simulink model "MTDC_MODEL"  (R2021a)
settings: Solver=ode1  StartTime=0.0  StopTime=3  FixedStep=2e-5  MaxStep=1e-5  RelTol=1e-5  EnableMultiTasking=on
InitFcn:
  | tau_iac=ts_G_iac/4;                                         %Current loop speed
  | wAC=1/tau_iac;                                              %Frequency
  | L1AC=wAC/s;                                                 %Open loop IMC (L) transfer function to obtain a first order after closing the loop
  | Kp_AC=wAC*(Lg_1+La_1/2);                                    %Proportional constant of the controller
  | Ki_AC=wAC*(Rg_1+Ra_1/2);                                    %Integral constant of the controller
  | C_IMC_AC=(Kp_AC*s+Ki_AC)/s;                                 %IMC designed PI controller transfer function
  | TAC=minreal((C_IMC_AC)*G_iac/(1+(C_IMC_AC)*G_iac));         %Closed loop transfer function
  | 
  | tau_Pac=ts_G_P/4;
  | D = TAC*U_ll1;
  | [C_pi,info] = pidtune(D,'PI',1/tau_Pac);
  | Ki_P = C_pi.Ki;
  | 
  | tau_Qac=ts_G_Q/4;
  | [C_piq,info] = pidtune(D,'PI',1/tau_Qac);
  | Ki_Q = C_piq.Ki;
  | 
  | 
  | tau_isum=ts_G_isum/4;                                        %Current loop speed
  | wsum=1/tau_isum;                                             %Frequency
  | L1AC=wsum/s;                                                 %Open loop IMC (L) transfer function to obtain a first order after closing the loop
  | Kp_sum=wsum*(2*La_1);                                        %Proportional constant of the controller
  | Ki_sum=wsum*(2*Ra_1);                                        %Integral constant of the controller
  | C_IMC_sum=(Kp_sum*s+Ki_sum)/s;                               %IMC designed PI controller transfer function
  | 
  | Kp_sum_PR = wc*(2*La_1);
  | Ki_sum_PR = wc*(2*Ra_1);
  | PR = (Kp_sum_PR*s^2 + 2*wc*(Kp_sum_PR+Ki_sum_PR)*s +Kp_sum_PR*w0^2)/(s^2+2*wc*s+w0^2);
  | 
  | 
  | %Energy reference for a converter arm (sum of all the submodule energies)
  | ArmEnergyRef=1/2*Carm*ArmVoltageRef^2;                      %Energy reference for a converter leg
  | LegEnergy=ArmEnergyRef*2;                                   %References for the controllers (DC side)
  | TotalEnergyRef=ArmEnergyRef*6;                              %Reference of the total energy of the converter
  | EnergyDiffabRef=0;                                          %Reference for the energy difference between legs a and b
  | EnergyDiffacRef=0;                                          %Reference for the energy difference between legs b and c
  | 
  | %References for the controllers (AC side)
  | EnergyDiffUpLowRefa=0;                                      %Reference for the energy difference upper and lower arms of phase a
  | EnergyDiffUpLowRefb=0;                                      %Reference for the energy difference upper and lower arms of phase b
  | EnergyDiffUpLowRefc=0;                                      %Reference for the energy difference upper and lower arms of phase c
  |                                                             %Controller design
  | Kpenergy=50;                                                %Proportional gain
  | Kienergy=20;                                                %Integral gain
  | 
  | Kpenergyt=50;                                               %Proportional gain
  | Kienergyt=20;                                               %Integral gain
  | 
  | Q=3;
  | wn=50*2*pi;                                                 %Frequency to eliminate 50 Hz
  | N_50 = tf([1 0 wn^2],[1 2*wn/Q wn^2]);                       %Notch filter 1 design
  | wn=100*2*pi;                                                %Frequency to eliminate 100 Hz
  | N_100 = tf([1 0 wn^2],[1 2*wn/Q wn^2]);                      %Notch filter 2 design
  | Notch=N_50*N_100;                                            %Combination of both notch filters
  | 
  | Ibasedc1= 1000e6/640e3;                 %Nominal current peak DC
  | IsaturationinnerDC1=1.1*Ibasedc1/3;  %Saturation of the DC inner current
  | IsaturationinnerAC1=0.45*Ibasedc1/3; %0.45  %Saturation of the inner current (why edu used 10% - FYI I changed it to 45%)
  | 
  | 
  | ... (+30 lines)
values from neighbouring files (symbols this model uses):
  ArmVoltageRef = 640e3    (= 640000)    [MMC_PARAMETERS.m]
  Cap = 9.5e-3    (= 0.0095)    [MMC_PARAMETERS.m]
  Carm = Cap/N    (= 2.375e-05)    [MMC_PARAMETERS.m]
  f_grid = 50    [MMC_PARAMETERS.m]
  La_1 = 0.15*Zbase_1/2/pi/50    (= 0.0488923985178)    [MMC_PARAMETERS.m]
  Lg_1 = 0.18*Zbase_1/2/pi/50    (= 0.0586708782214)    [MMC_PARAMETERS.m]
  N = 400    [MMC_PARAMETERS.m]
  Ra_1 = 0.01*Zbase_1    (= 1.024)    [MMC_PARAMETERS.m]
  Rg_1 = 0.005*Zbase_1    (= 0.512)    [MMC_PARAMETERS.m]
  S_1 = 1000e6    (= 1000000000)    [MMC_PARAMETERS.m]
  U_ll1 = 320e3    (= 320000)    [MMC_PARAMETERS.m]
  Vdc = 640e3    (= 640000)    [MMC_PARAMETERS.m]
  Vpeak_d1 = U_pnpeak1    [MMC_PARAMETERS.m]
  w0 = 2*pi*50    (= 314.159265359)    [MMC_PARAMETERS.m]
undefined symbols (not defined in the file or in its folder): Kp_Pac, lenght
libraries: spsSeriesRLCBranchLib x80, spsCurrentMeasurementLib x64, spsControlledVoltageSourceLib x36, pid_lib x32, spsVoltageMeasurementLib x32, spsControlledCurrentSourceLib x24, spsParallelRLCBranchLib x20, spsGroundLib x10, powerlib_extras x4, spsDCVoltageSourceLib x4, spspowerguiLib x1
(part 4 of 9)

== system MTDC_MODEL/GRID1+MMC1/Equivalent arm upper-b ==
  note: Power_ub
  vub : Inport
  Controlled Current Source : spsControlledCurrentSourceLib/Controlled Current Source  Initialize=on  Source_Type=AC  Amplitude=0  Phase=0  Frequency=0  Measurements=None
  Controlled Voltage Source7 : spsControlledVoltageSourceLib/Controlled Voltage Source  Initialize=on  Source_Type=AC  Amplitude=Vdc/2  Phase=0  Frequency=0  Measurements=None
  Current Measurement4 : spsCurrentMeasurementLib/Current Measurement  PhasorSimulation=off  OutputType=Complex  PSBequivalent=0
  Divide1 : Product  Inputs=**
  Divide2 : Product  Inputs=*/
  Filtered Upper arm A instananeous power1 : Scope
  Gain : Gain  Gain=1e6
  Series RLC Branch2 : spsSeriesRLCBranchLib/Series RLC Branch  LConnTagsString=__new0  RConnTagsString=__new0  BranchType=C  Resistance=Ra_1  Inductance=La_1  SetiL0=on  InitialCurrent=0  Capacitance=Cap/N  Setx0=on  InitialVoltage=640e3  Measurements=None
  Transfer Fcn : TransferFcn  Denominator=[1 1]
  Upper arm A instananeous power : Scope
  Voltage Measurement : spsVoltageMeasurementLib/Voltage Measurement  PhasorSimulation=off  OutputType=Complex  PSBequivalent=0
  Conn1 : PMIOPort  Side=Right
  Conn2 : PMIOPort  Port=2  Side=Left
  v_sum_ub : Outport
  wires:
  vub/1 -> Divide1/1, Controlled Voltage Source7/1  "vub"
  Voltage Measurement/1 -> v_sum_ub/1, Divide2/2
  Divide2/1 -> Controlled Current Source/1
  Divide1/1 -> Upper arm A instananeous power/1, Transfer Fcn/1, Divide2/1
  Current Measurement4/1 -> Divide1/2  "iub"
  Transfer Fcn/1 -> Gain/1
  Gain/1 -> Filtered Upper arm A instananeous power1/1
  connections:
  Controlled Voltage Source7/RConn1 -- Conn1/RConn1
  Voltage Measurement/LConn1 -- Series RLC Branch2/LConn1 -- Controlled Current Source/RConn1
  Controlled Current Source/LConn1 -- Series RLC Branch2/RConn1 -- Voltage Measurement/LConn2
  Current Measurement4/LConn1 -- Controlled Voltage Source7/LConn1
  Conn2/RConn1 -- Current Measurement4/RConn1

== system MTDC_MODEL/GRID1+MMC1/Equivalent arm upper-c ==
  note: Power_uc
  vuc : Inport
  Controlled Current Source : spsControlledCurrentSourceLib/Controlled Current Source  Initialize=on  Source_Type=AC  Amplitude=0  Phase=0  Frequency=0  Measurements=None
  Controlled Voltage Source7 : spsControlledVoltageSourceLib/Controlled Voltage Source  Initialize=on  Source_Type=AC  Amplitude=Vdc/2  Phase=0  Frequency=0  Measurements=None
  Current Measurement4 : spsCurrentMeasurementLib/Current Measurement  PhasorSimulation=off  OutputType=Complex  PSBequivalent=0
  Divide1 : Product  Inputs=**
  Divide2 : Product  Inputs=*/
  Filtered Upper arm A instananeous power1 : Scope
  Gain : Gain  Gain=1e6
  Series RLC Branch2 : spsSeriesRLCBranchLib/Series RLC Branch  LConnTagsString=__new0  RConnTagsString=__new0  BranchType=C  Resistance=Ra_1  Inductance=La_1  SetiL0=on  InitialCurrent=0  Capacitance=Cap/N  Setx0=on  InitialVoltage=640e3  Measurements=None
  Transfer Fcn : TransferFcn  Denominator=[1 1]
  Upper arm A instananeous power : Scope
  Voltage Measurement : spsVoltageMeasurementLib/Voltage Measurement  PhasorSimulation=off  OutputType=Complex  PSBequivalent=0
  Conn1 : PMIOPort  Side=Right
  Conn2 : PMIOPort  Port=2  Side=Left
  v_sum_uc : Outport
  wires:
  vuc/1 -> Divide1/1, Controlled Voltage Source7/1  "vuc"
  Voltage Measurement/1 -> v_sum_uc/1, Divide2/2
  Divide2/1 -> Controlled Current Source/1
  Divide1/1 -> Upper arm A instananeous power/1, Transfer Fcn/1, Divide2/1
  Current Measurement4/1 -> Divide1/2  "iuc"
  Transfer Fcn/1 -> Gain/1
  Gain/1 -> Filtered Upper arm A instananeous power1/1
  connections:
  Controlled Voltage Source7/RConn1 -- Conn1/RConn1
  Voltage Measurement/LConn1 -- Series RLC Branch2/LConn1 -- Controlled Current Source/RConn1
  Controlled Current Source/LConn1 -- Series RLC Branch2/RConn1 -- Voltage Measurement/LConn2
  Current Measurement4/LConn1 -- Controlled Voltage Source7/LConn1
  Conn2/RConn1 -- Current Measurement4/RConn1

== system MTDC_MODEL/GRID1+MMC1/Feedforward calculation ==
  vzabc : Inport
  isabc : Inport  Port=2
  Demux1 : Demux  Outputs=3
  First order filter1 : Subsystem
  Mux2 : Mux  Inputs=2
  PI10 : TransferFcn  Numerator=[Notch.num{1}]  Denominator=[Notch.den{1}]
  PI9 : TransferFcn  Numerator=[Notch.num{1}]  Denominator=[Notch.den{1}]
  Product5 : Product
  Scope3 : Scope
  Sum15 : Sum  Inputs=|+-
  Sum39 : Sum  Inputs=|+-
  Sum5 : Sum  Inputs=+++
  Pt : Outport  VectorParamsAs1DForOutWhenUnconnected=off
  Pab : Outport  Port=2  VectorParamsAs1DForOutWhenUnconnected=off
  Pac : Outport  Port=3  VectorParamsAs1DForOutWhenUnconnected=off
  wires:
  Demux1/3 -> Sum39/2, Sum5/3
  Demux1/2 -> Sum15/2, Sum5/2
  Demux1/1 -> Sum15/1, Sum39/1, Sum5/1
  vzabc/1 -> Product5/1
  Sum15/1 -> Pab/1, PI9/1  "Pa-Pb"
  Sum39/1 -> Pac/1, PI10/1  "Pb-Pc"
  Product5/1 -> First order filter1/1(In1)
  First order filter1/1(Out1) -> Demux1/1
  isabc/1 -> Product5/2
  Sum5/1 -> Pt/1
  Mux2/1 -> Scope3/1
  PI9/1 -> Mux2/1
  PI10/1 -> Mux2/2

== system MTDC_MODEL/GRID1+MMC1/Grid3 ==
  Constant : Constant
  Constant1 : Constant  Value=f_grid
  Constant{2,5..7,20} (5 alike) : Constant  Value=0
  Constant21 : Constant  Value=-2*pi/3
  Constant22 : Constant  Value=2*pi/3
  Constant8 : Constant  Value=2*pi/3
  Constant9 : Constant  Value=-2*pi/3
  Gain1 : Gain  Gain=2*pi
  Gain{2..3,6,8} (4 alike) : Gain  Gain=Vpeak_d1
  Gain4 : Gain  Gain=0
  Gain5 : Gain  Gain=0
  Gain7 : Gain  Gain=0
  Integrator{1..3,8..10} (6 alike) : Integrator
  Sum{1..12} (12 alike) : Sum  Inputs=|++
  Trigonometric Function{1..3,6..8} (6 alike) : Trigonometry  Operator=cos
  vza : Outport
  vzb : Outport  Port=2
  vzc : Outport  Port=3
  thetareal : Outport  Port=4
  vpos : Outport  Port=5
  wires:
  Sum12/1 -> vzc/1
  Sum11/1 -> vzb/1
  Sum10/1 -> vza/1
  Constant6/1 -> Sum12/2
  Constant5/1 -> Sum11/2
  Constant2/1 -> Sum10/2
  Sum6/1 -> Sum12/1
  Sum5/1 -> Sum11/1
  Sum4/1 -> Sum10/1
  Gain5/1 -> Sum6/2
  Gain4/1 -> Sum5/2
  Gain7/1 -> Sum4/2
  Trigonometric Function2/1 -> Gain4/1
  Trigonometric Function3/1 -> Gain5/1
  Sum3/1 -> Trigonometric Function1/1
  Constant9/1 -> Sum2/2
  Integrator1/1 -> Sum2/1
  Constant8/1 -> Sum1/2
  Integrator2/1 -> Sum3/1
  Gain1/1 -> Integrator9/1, Integrator8/1, Integrator10/1, Integrator2/1, Integrator1/1, Integrator3/1
  Sum1/1 -> Trigonometric Function2/1
  Constant7/1 -> Sum3/2
  Trigonometric Function1/1 -> Gain7/1
  Integrator3/1 -> Sum1/1
  Sum2/1 -> Trigonometric Function3/1
  Gain3/1 -> Sum6/1
  Gain2/1 -> Sum5/1
  Gain8/1 -> Sum4/1
  Trigonometric Function7/1 -> Gain2/1
  Trigonometric Function8/1 -> Gain3/1
  Constant1/1 -> Gain1/1
  Sum9/1 -> thetareal/1, Trigonometric Function6/1
  Constant22/1 -> Sum8/2
  Integrator10/1 -> Sum8/1
  Constant21/1 -> Sum7/2
  Integrator8/1 -> Sum9/1
  Sum7/1 -> Trigonometric Function7/1
  Constant20/1 -> Sum9/2
  Trigonometric Function6/1 -> Gain8/1
  Integrator9/1 -> Sum7/1
  Sum8/1 -> Trigonometric Function8/1
  Constant/1 -> Gain6/1
  Gain6/1 -> vpos/1

== system MTDC_MODEL/GRID1+MMC1/Isum_AC_Ref_Cal ==
  note: negative sequence
  note: positive sequence
  Pdiff_arm_a_Ref : Inport
  Pdiff_arm_b_Ref : Inport  Port=2
  Pdiff_arm_c_Ref : Inport  Port=3
  Clarke : Inport  Port=4
  v_g_pos : Inport  Port=5
  theta : Inport  Port=6
  Constant5 : Constant  Value=0
  Constant7 : Constant  Value=0
  "DIFFERENT_REF_CALC_METHODS " : Subsystem
  Demux2 : Demux
  Demux3 : Demux  Outputs=3
  Display : Display
  Gain1 : Gain  Gain=1/S_1
  Gain10 : Gain  Gain=-1
  Gain11 : Gain  Gain=sqrt(2)
  Gain19 : Gain  Gain=S_1/(U_ll1)
  Gain2 : Gain  Gain=1/S_1
  Gain3 : Gain  Gain=1/S_1
  Matrix Multiply{,1..2,6} (4 alike) : Product  Multiplication=Matrix(*)
  Mux28 : Mux  Inputs=2
  Mux57 : Mux  Inputs=3
  Mux6 : Mux
  Mux8 : Mux  Inputs=2
  Mux9 : Mux  Inputs=2
  Rotation4 : Subsystem
  Scope4 : Scope
  Sum7 : Sum  Inputs=+|+
  i_albe_AC : Outport  VectorParamsAs1DForOutWhenUnconnected=off
  wires:
  Mux57/1 -> Matrix Multiply1/2
  Matrix Multiply1/1 -> Matrix Multiply2/2  "P_al; P_be; P_0"
  Mux6/1 -> Gain19/1
  Constant7/1 -> Mux6/4
  Matrix Multiply2/1 -> Demux3/1
  Demux3/1 -> Mux6/1  "Isum_neg"
  Demux3/2 -> Gain10/1  "-Isum_neg"
  Gain10/1 -> Mux6/2
  Demux3/3 -> Mux6/3  "Isum_pos"
  Pdiff_arm_a_Ref/1 -> Gain3/1
  Pdiff_arm_b_Ref/1 -> Gain2/1
  Pdiff_arm_c_Ref/1 -> Gain1/1
  Clarke/1 -> Matrix Multiply1/1
  "DIFFERENT_REF_CALC_METHODS "/1(Initial Approach) -> Matrix Multiply2/1, Display/1
  Gain3/1 -> Mux57/1
  Gain2/1 -> Mux57/2
  Gain1/1 -> Mux57/3
  Gain19/1 -> Gain11/1
  [R] -> Matrix Multiply/1
  [iR] -> Matrix Multiply6/1
  Constant5/1 -> Mux28/2
  Gain11/1 -> Scope4/1, Demux2/1
  Matrix Multiply/1 -> Sum7/1
  Mux28/1 -> i_albe_AC/1
  Matrix Multiply6/1 -> Sum7/2
  Demux2/3 -> Mux9/1
  Demux2/2 -> Mux8/2
  Sum7/1 -> Mux28/1
  Demux2/1 -> Mux8/1
  Demux2/4 -> Mux9/2
  Rotation4/2(R) -> [R]
  Rotation4/1(iR) -> [iR]
  theta/1 -> Rotation4/1(angle)
  Mux8/1 -> Matrix Multiply/2
  Mux9/1 -> Matrix Multiply6/2
  v_g_pos/1 -> "DIFFERENT_REF_CALC_METHODS "/1(v_g_pos)

== system MTDC_MODEL/GRID1+MMC1/Modulation ==
  vdiffabc : Inport
  vsumabc : Inport  Port=2
  Constant12 : Constant  Value=[-1 0 0 1/2 0 0;0 -1 0 0 1/2 0 ;0 0 -1 0 0 1/2;1 0 0 1/2 0 0;0 1 0 0 1/2 0;0 0 1 0 0 1/2]  SampleTime=-1
  Demux3 : Demux  Outputs=6
  Gain1 : Gain  Gain=-1
  Matrix Multiply1 : Product  Multiplication=Matrix(*)
  Mux12 : Mux  Inputs=2
  Mux17 : Mux  Inputs=3
  Mux19 : Mux  Inputs=3
  vuabc : Outport
  vlabc : Outport  Port=2
  wires:
  Constant12/1 -> Matrix Multiply1/1
  Mux12/1 -> Matrix Multiply1/2
  vdiffabc/1 -> Mux12/1
  Matrix Multiply1/1 -> Demux3/1
  Gain1/1 -> Mux12/2
  vsumabc/1 -> Gain1/1
  Mux17/1 -> vuabc/1
  Mux19/1 -> vlabc/1
  Demux3/3 -> Mux17/3
  Demux3/2 -> Mux17/2
  Demux3/1 -> Mux17/1
  Demux3/6 -> Mux19/3
  Demux3/5 -> Mux19/2
  Demux3/4 -> Mux19/1

== system MTDC_MODEL/GRID1+MMC1/Park//nPark2 ==
  theta : Inport
  Constant1 : Constant  Value=1/2  SampleTime=0
  Constant2 : Constant  Value=1/2  SampleTime=0
  Constant3 : Constant  Value=1/2  SampleTime=0
  Constant4 : Constant  Value=2*pi/3  SampleTime=0
  Constant5 : Constant  SampleTime=0
  Constant6 : Constant  SampleTime=0
  Constant7 : Constant  SampleTime=0
  Gain7 : Gain  Gain=2/3
  Matrix Concatenate1 : Concatenate  NumInputs=3  Mode=Multidimensional array  ConcatenateDimension=2
  Matrix Concatenate2 : Concatenate  NumInputs=3  Mode=Multidimensional array  ConcatenateDimension=2
  Mux{1..6} (6 alike) : Mux  Inputs=3
  Sum1 : Sum  Inputs=|++
  Sum2 : Sum  Inputs=|+-
  Trigonometric Function : Trigonometry  Operator=cos
  Trigonometric Function1 : Trigonometry
  Trigonometric Function2 : Trigonometry  Operator=cos
  Trigonometric Function3 : Trigonometry
  Trigonometric Function4 : Trigonometry  Operator=cos
  Trigonometric Function5 : Trigonometry
  T : Outport
  "nT " : Outport  Port=2
  wires:
  Matrix Concatenate2/1 -> "nT "/1
  Gain7/1 -> T/1
  theta/1 -> Trigonometric Function1/1, Trigonometric Function/1, Sum2/1, Sum1/1
  Mux6/1 -> Matrix Concatenate2/2
  Mux5/1 -> Matrix Concatenate2/1
  Matrix Concatenate1/1 -> Gain7/1
  Mux3/1 -> Matrix Concatenate1/3
  Mux1/1 -> Matrix Concatenate1/2
  Mux2/1 -> Matrix Concatenate1/1
  Trigonometric Function5/1 -> Mux3/2, Mux6/3
  Trigonometric Function4/1 -> Mux5/3, Mux3/1
  Trigonometric Function3/1 -> Mux1/2, Mux6/2
  Trigonometric Function2/1 -> Mux1/1, Mux5/2
  Trigonometric Function1/1 -> Mux6/1, Mux2/2
  Trigonometric Function/1 -> Mux5/1, Mux2/1
  Constant4/1 -> Sum1/2, Sum2/2
  Sum1/1 -> Trigonometric Function5/1, Trigonometric Function4/1
  Sum2/1 -> Trigonometric Function3/1, Trigonometric Function2/1
  Constant1/1 -> Mux2/3
  Constant2/1 -> Mux1/3
  Constant3/1 -> Mux3/3
  Constant5/1 -> Mux4/1
  Constant6/1 -> Mux4/2
  Constant7/1 -> Mux4/3
  Mux4/1 -> Matrix Concatenate2/3

== system MTDC_MODEL/GRID1+MMC1/Power_calculation ==
  Pua : Inport
  Pla : Inport  Port=2
  Pub : Inport  Port=3
  Plb : Inport  Port=4
  Puc : Inport  Port=5
  Plc : Inport  Port=6
  Sum : Sum
  Sum1 : Sum
  Sum2 : Sum
  Sum3 : Sum  Inputs=+++
  Sum{4..8} (5 alike) : Sum  Inputs=+-
  Pab : Outport
  Pac : Outport  Port=2
  Pt : Outport  Port=3
  Pula : Outport  Port=4
  Pulb : Outport  Port=5
  Pulc : Outport  Port=6
  wires:
  Sum2/1 -> Sum3/3, Sum7/2
  Sum3/1 -> Pt/1
  Sum/1 -> Sum3/2, Sum7/1, Sum6/1
  Sum1/1 -> Sum3/1, Sum6/2
  Pla/1 -> Sum4/2, Sum/2
  Sum6/1 -> Pab/1
  Sum7/1 -> Pac/1
  Pua/1 -> Sum4/1, Sum/1
  Sum4/1 -> Pula/1
  Sum5/1 -> Pulb/1
  Pub/1 -> Sum5/1, Sum1/1
  Plb/1 -> Sum5/2, Sum1/2
  Plc/1 -> Sum8/2, Sum2/2
  Puc/1 -> Sum2/1, Sum8/1
  Sum8/1 -> Pulc/1

== system MTDC_MODEL/GRID1+MMC1/Subsystem1 ==
  Uuabc : Inport
  Iuabc : Inport  Port=2
  Ulabc : Inport  Port=3
  Ilabc : Inport  Port=4
  Demux{,2,4,6} (4 alike) : Demux  Outputs=3
  Product{,1..5} (6 alike) : Product
  Pua : Outport
  Pub : Outport  Port=2
  Puc : Outport  Port=3
  Pla : Outport  Port=4
  Plb : Outport  Port=5
  Plc : Outport  Port=6
  wires:
  Demux6/2 -> Product4/2
  Demux2/2 -> Product1/2
  Demux6/3 -> Product5/2
  Ulabc/1 -> Demux4/1
  Demux2/1 -> Product/2
  Uuabc/1 -> Demux/1
  Demux2/3 -> Product2/2
  Demux6/1 -> Product3/2
  Demux/1 -> Product/1
  Product5/1 -> Plc/1
  Demux4/3 -> Product5/1
  Demux4/2 -> Product4/1
  Demux4/1 -> Product3/1
  Ilabc/1 -> Demux6/1
  Demux/3 -> Product2/1
  Demux/2 -> Product1/1
  Product/1 -> Pua/1
  Product1/1 -> Pub/1
  Product3/1 -> Pla/1
  Product4/1 -> Plb/1
  Product2/1 -> Puc/1
  Iuabc/1 -> Demux2/1

== system MTDC_MODEL/GRID1+MMC1/Voltage calculation ==
  vus_a : Inport
  vus_b : Inport  Port=2
  vus_c : Inport  Port=3
  vls_a : Inport  Port=4
  vls_b : Inport  Port=5
  vls_c : Inport  Port=6
  Mux11 : Mux  Inputs=3
  Sum : Sum  Inputs=|++
  Sum10 : Sum  Inputs=|++
  Sum11 : Sum  Inputs=+-|
  Sum12 : Sum  Inputs=+++
  Sum2 : Sum  Inputs=+-|
  Sum9 : Sum  Inputs=|++
  v_total_abc : Outport
  V_diff_ab : Outport  Port=2
  V_diff_ac : Outport  Port=3
  V_t_MMC : Outport  Port=4
  wires:
  vus_c/1 -> Sum10/1
  Sum/1 -> Sum11/1, Mux11/1, Sum12/1, Sum2/1  "v_total_a"
  vls_c/1 -> Sum10/2
  Mux11/1 -> v_total_abc/1
  Sum11/1 -> V_diff_ab/1  "V_diff_ab"
  vus_a/1 -> Sum/1
  Sum10/1 -> Sum2/2, Mux11/3, Sum12/3  "v_total_c"
  Sum9/1 -> Sum11/2, Mux11/2, Sum12/2  "v_total_b"
  vls_b/1 -> Sum9/2
  Sum2/1 -> V_diff_ac/1  "V_diff_ac"
  vus_b/1 -> Sum9/1
  Sum12/1 -> V_t_MMC/1  "V_t_MMC"
  vls_a/1 -> Sum/2

== system MTDC_MODEL/GRID1+MMC1/Voltage calculation1 ==
  vus_a : Inport
  vus_b : Inport  Port=2
  vus_c : Inport  Port=3
  vls_a : Inport  Port=4
  vls_b : Inport  Port=5
  vls_c : Inport  Port=6
  Sum : Sum  Inputs=|+-
  Sum10 : Sum  Inputs=|+-
  Sum9 : Sum  Inputs=|+-
  v_total_a : Outport
  v_total_b : Outport  Port=2
  v_total_c : Outport  Port=3
  wires:
  vls_a/1 -> Sum/2
  vus_b/1 -> Sum9/1
  vls_b/1 -> Sum9/2
  Sum9/1 -> v_total_b/1  "v_total_b"
  Sum10/1 -> v_total_c/1  "v_total_c"
  vus_a/1 -> Sum/1
  vls_c/1 -> Sum10/2
  Sum/1 -> v_total_a/1  "v_total_a"
  vus_c/1 -> Sum10/1

== system MTDC_MODEL/GRID1+MMC1/vsum Calculation ==
  Inner_current_refs : Inport
  i_uabc : Inport  Port=2
  i_labc : Inport  Port=3
  irefabcDC : Inport  Port=4
  Constant : Constant  Value=640e3
  Constant15 : Constant  Value="[1  0 0 1 0 0;0 1 0 0 1 0 ;0 0 1 0 0 1]"  SampleTime=-1
  Demux{1..4,7} (5 alike) : Demux  Outputs=3
  Gain1 : Gain  Gain=1/2
  Gain2 : Gain  Gain=1/2
  Matrix Multiply{2,10,13,18} (4 alike) : Product  Multiplication=Matrix(*)
  Memory : Memory
  Memory1 : Memory
  Memory2 : Memory  InitialCondition=-Vdc
  Mux13 : Mux  Inputs=3
  Mux18 : Mux  Inputs=2
  PR Controller1 : Subsystem
  PR Controller2 : Subsystem
  PR Controller3 : Subsystem
  Scope : Scope
  Scope1 : Scope  NumInputPorts=3
  Sum1 : Sum  Inputs=++|
  Sum{3,5..6,11} (4 alike) : Sum  Inputs=|+-
  Sum13 : Sum  Inputs=++|
  To File3 : ToFile  Filename=isumapi.mat  MatrixName=ans0006  SaveFormat=Timeseries
  vsumabc : Outport  VectorParamsAs1DForOutWhenUnconnected=off
  wires:
  Mux13/1 -> Matrix Multiply10/2
  Gain1/1 -> Matrix Multiply2/2
  Sum13/1 -> Demux7/1
  Demux3/1 -> Sum5/2
  Demux7/3 -> Sum6/1
  Demux7/2 -> Sum3/1
  Demux3/3 -> Sum6/2
  PR Controller1/1(v) -> Memory/1
  Sum5/1 -> PR Controller1/1(e)
  Sum6/1 -> PR Controller3/1(e)
  Sum3/1 -> PR Controller2/1(e)
  PR Controller2/1(v) -> Memory1/1
  Demux3/2 -> Sum3/2
  PR Controller3/1(v) -> Sum11/1
  Sum11/1 -> Memory2/1
  Matrix Multiply18/1 -> Sum13/2
  Constant/1 -> Sum11/2
  irefabcDC/1 -> Matrix Multiply18/2
  Mux18/1 -> Matrix Multiply13/2
  Constant15/1 -> Matrix Multiply13/1
  Matrix Multiply13/1 -> Gain1/1
  Demux7/1 -> Sum5/1
  Matrix Multiply2/1 -> Demux3/1
  [nC] -> Matrix Multiply10/1
  [Clarke] -> Matrix Multiply18/1
  [Clarke] -> Matrix Multiply2/1
  Matrix Multiply10/1 -> Demux1/1, vsumabc/1
  Memory/1 -> Mux13/1
  Memory1/1 -> Mux13/2
  Memory2/1 -> Scope/1, Mux13/3
  Inner_current_refs/1 -> Sum13/1
  i_labc/1 -> Demux4/1, Mux18/2
  Sum1/1 -> Gain2/1
  Gain2/1 -> To File3/1
  Demux4/1 -> Sum1/2
  Demux2/1 -> Sum1/1
  i_uabc/1 -> Demux2/1, Mux18/1
  Demux1/1 -> Scope1/1
  Demux1/2 -> Scope1/2
  Demux1/3 -> Scope1/3

== system MTDC_MODEL/GRID2+MMC2/Calculo Referencias ==
  P_ref : Inport
  P : Inport  Port=2
  Q_ref : Inport  Port=3
  Q : Inport  Port=4
  V_DC : Inport  Port=5
  Constant : Constant  Value=Vdc*1.004
  Constant1 : Constant  Value=sqrt(2)*1000*Vdc/(3*U_ll1)
  Gain : Gain  Gain=-1
  Gain1 : Gain  Gain=-1
  Gain2 : Gain
  PID Controller1 : pid_lib/PID Controller  Controller=I  Form=Parallel  TimeDomain=Continuous-time  UseExternalTs=off  SampleTime=1  IntegratorMethod=Forward Euler  FilterMethod=Forward Euler  ControllerParametersSource=internal  P=Kp_Pac  I=Ki_Q  D=0  UseFilter=on  N=100  TunerSelectOption=Transfer Function Based (PID Tuner App)  InitialConditionSource=internal  InitialConditionForIntegrator=0  InitialConditionForFilter=0  DifferentiatorICPrevScaledInput=0  ExternalReset=none  TrackingMode=off  Kt=1  LimitOutput=off  SatLimitsSource=internal  UpperSaturationLimit=inf  LowerSaturationLimit=-inf  LinearizeAsGain=on  AntiWindupMode=none  Kb=1  POutMin=[]  POutMax=[]  IOutMin=[]  IOutMax=[]  DOutMin=[]  DOutMax=[]  NOutMin=[]  NOutMax=[]  SumOutMin=[]  SumOutMax=[]  SaturationOutMin=[]  SaturationOutMax=[]  PParamMin=[]  PParamMax=[]  IParamMin=[]  IParamMax=[]  DParamMin=[]  DParamMax=[]  NParamMin=[]  NParamMax=[]  KbParamMin=[]  KbParamMax=[]  KtParamMin=[]  KtParamMax=[]  KbOutMin=[]  KbOutMax=[]  KtOutMin=[]  KtOutMax=[]  IntegratorOutMin=[]  IntegratorOutMax=[]  FilterOutMin=[]  FilterOutMax=[]  SumI1OutMin=[]  SumI1OutMax=[]  SumI2OutMin=[]  SumI2OutMax=[]  SumI3OutMin=[]  SumI3OutMax=[]  SumI4OutMin=[]  SumI4OutMax=[]  SumDOutMin=[]  SumDOutMax=[]  DifferentiatorOutMin=[]  DifferentiatorOutMax=[]  FilterDiffOutCoefMin=[]  FilterDiffOutCoefMax=[]  ReciprocalOutMin=[]  ReciprocalOutMax=[]  SumDenOutMin=[]  SumDenOutMax=[]  SumNumOutMin=[]  SumNumOutMax=[]  DivideOutMin=[]  DivideOutMax=[]  UdiffTsProdOutMin=[]  UdiffTsProdOutMax=[]  NTsProdOutMin=[]  NTsProdOutMax=[]  UintegralTsProdOutMin=[]  UintegralTsProdOutMax=[]  UngainTsProdOutMin=[]  UngainTsProdOutMax=[]  IntegratorContinuousStateAttributes=''  IntegratorStateMustResolveToSignalObject=off  IntegratorRTWStateStorageClass=Auto  FilterContinuousStateAttributes=''  FilterStateMustResolveToSignalObject=off  FilterRTWStateStorageClass=Auto  ParallelPVariant=Disabled  IdealPVariant=Disabled  IVariant=InternalParameters  DVariant=Disabled  IntegratorVariant=Continuous  SatVariant=Disabled  AWVariant=Passthrough  PCopyVariant=Disabled  TRVariant=Disabled  FdbkBlocksVariant=Forward  IdealPFdbkVariant=Disabled  SatFdbkVariant=Disabled  DerivativeFilterVariant=Disabled  NVariant=Disabled  NCopyVariant=Disabled_SignalSpec  FilterICVariant=Disabled  IntegratorICVariant=InternalICs  ExternalResetVariant=Disabled  TRSumVariant=Passthrough  SumFdbkVariant=Disabled  SumVariant=Passthrough_I  TsampFilterVariant=InternalTs  TsampNgainVariant=Passthrough  TsampIntegralVariant=Passthrough  ExternalSaturationOutDataTypeStr=Inherit: Same as second input
  PID Controller2 : pid_lib/PID Controller  Controller=PI  Form=Parallel  TimeDomain=Continuous-time  UseExternalTs=off  SampleTime=1  IntegratorMethod=Forward Euler  FilterMethod=Forward Euler  ControllerParametersSource=internal  P=7.77e-5  I=7.094e-6  D=0  UseFilter=on  N=100  TunerSelectOption=Frequency Response Based  InitialConditionSource=internal  InitialConditionForIntegrator=0  InitialConditionForFilter=0  DifferentiatorICPrevScaledInput=0  ExternalReset=none  TrackingMode=off  Kt=1  LimitOutput=off  SatLimitsSource=internal  UpperSaturationLimit=inf  LowerSaturationLimit=-inf  LinearizeAsGain=on  AntiWindupMode=none  Kb=1  POutMin=[]  POutMax=[]  IOutMin=[]  IOutMax=[]  DOutMin=[]  DOutMax=[]  NOutMin=[]  NOutMax=[]  SumOutMin=[]  SumOutMax=[]  SaturationOutMin=[]  SaturationOutMax=[]  PParamMin=[]  PParamMax=[]  IParamMin=[]  IParamMax=[]  DParamMin=[]  DParamMax=[]  NParamMin=[]  NParamMax=[]  KbParamMin=[]  KbParamMax=[]  KtParamMin=[]  KtParamMax=[]  KbOutMin=[]  KbOutMax=[]  KtOutMin=[]  KtOutMax=[]  IntegratorOutMin=[]  IntegratorOutMax=[]  FilterOutMin=[]  FilterOutMax=[]  SumI1OutMin=[]  SumI1OutMax=[]  SumI2OutMin=[]  SumI2OutMax=[]  SumI3OutMin=[]  SumI3OutMax=[]  SumI4OutMin=[]  SumI4OutMax=[]  SumDOutMin=[]  SumDOutMax=[]  DifferentiatorOutMin=[]  DifferentiatorOutMax=[]  FilterDiffOutCoefMin=[]  FilterDiffOutCoefMax=[]  ReciprocalOutMin=[]  ReciprocalOutMax=[]  SumDenOutMin=[]  SumDenOutMax=[]  SumNumOutMin=[]  SumNumOutMax=[]  DivideOutMin=[]  DivideOutMax=[]  UdiffTsProdOutMin=[]  UdiffTsProdOutMax=[]  NTsProdOutMin=[]  NTsProdOutMax=[]  UintegralTsProdOutMin=[]  UintegralTsProdOutMax=[]  UngainTsProdOutMin=[]  UngainTsProdOutMax=[]  IntegratorContinuousStateAttributes=''  IntegratorStateMustResolveToSignalObject=off  IntegratorRTWStateStorageClass=Auto  FilterContinuousStateAttributes=''  FilterStateMustResolveToSignalObject=off  FilterRTWStateStorageClass=Auto  ParallelPVariant=InternalParameters  IdealPVariant=Disabled  IVariant=InternalParameters  DVariant=Disabled  IntegratorVariant=Continuous  SatVariant=Disabled  AWVariant=Passthrough  PCopyVariant=Disabled  TRVariant=Disabled  FdbkBlocksVariant=Forward  IdealPFdbkVariant=Disabled  SatFdbkVariant=Disabled  DerivativeFilterVariant=Disabled  NVariant=Disabled  NCopyVariant=Disabled_SignalSpec  FilterICVariant=Disabled  IntegratorICVariant=InternalICs  ExternalResetVariant=Disabled  TRSumVariant=Passthrough  SumFdbkVariant=Disabled  SumVariant=Sum_PI  TsampFilterVariant=InternalTs  TsampNgainVariant=Passthrough  TsampIntegralVariant=Passthrough  ExternalSaturationOutDataTypeStr=Inherit: Same as second input
  PID Controller4 : pid_lib/PID Controller  Controller=I  Form=Parallel  TimeDomain=Continuous-time  UseExternalTs=off  SampleTime=1  IntegratorMethod=Forward Euler  FilterMethod=Forward Euler  ControllerParametersSource=internal  P=Kp_Pac  I=Ki_P  D=0  UseFilter=on  N=100  TunerSelectOption=Transfer Function Based (PID Tuner App)  InitialConditionSource=internal  InitialConditionForIntegrator=0  InitialConditionForFilter=0  DifferentiatorICPrevScaledInput=0  ExternalReset=none  TrackingMode=off  Kt=1  LimitOutput=off  SatLimitsSource=internal  UpperSaturationLimit=inf  LowerSaturationLimit=-inf  LinearizeAsGain=on  AntiWindupMode=none  Kb=1  POutMin=[]  POutMax=[]  IOutMin=[]  IOutMax=[]  DOutMin=[]  DOutMax=[]  NOutMin=[]  NOutMax=[]  SumOutMin=[]  SumOutMax=[]  SaturationOutMin=[]  SaturationOutMax=[]  PParamMin=[]  PParamMax=[]  IParamMin=[]  IParamMax=[]  DParamMin=[]  DParamMax=[]  NParamMin=[]  NParamMax=[]  KbParamMin=[]  KbParamMax=[]  KtParamMin=[]  KtParamMax=[]  KbOutMin=[]  KbOutMax=[]  KtOutMin=[]  KtOutMax=[]  IntegratorOutMin=[]  IntegratorOutMax=[]  FilterOutMin=[]  FilterOutMax=[]  SumI1OutMin=[]  SumI1OutMax=[]  SumI2OutMin=[]  SumI2OutMax=[]  SumI3OutMin=[]  SumI3OutMax=[]  SumI4OutMin=[]  SumI4OutMax=[]  SumDOutMin=[]  SumDOutMax=[]  DifferentiatorOutMin=[]  DifferentiatorOutMax=[]  FilterDiffOutCoefMin=[]  FilterDiffOutCoefMax=[]  ReciprocalOutMin=[]  ReciprocalOutMax=[]  SumDenOutMin=[]  SumDenOutMax=[]  SumNumOutMin=[]  SumNumOutMax=[]  DivideOutMin=[]  DivideOutMax=[]  UdiffTsProdOutMin=[]  UdiffTsProdOutMax=[]  NTsProdOutMin=[]  NTsProdOutMax=[]  UintegralTsProdOutMin=[]  UintegralTsProdOutMax=[]  UngainTsProdOutMin=[]  UngainTsProdOutMax=[]  IntegratorContinuousStateAttributes=''  IntegratorStateMustResolveToSignalObject=off  IntegratorRTWStateStorageClass=Auto  FilterContinuousStateAttributes=''  FilterStateMustResolveToSignalObject=off  FilterRTWStateStorageClass=Auto  ParallelPVariant=Disabled  IdealPVariant=Disabled  IVariant=InternalParameters  DVariant=Disabled  IntegratorVariant=Continuous  SatVariant=Disabled  AWVariant=Passthrough  PCopyVariant=Disabled  TRVariant=Disabled  FdbkBlocksVariant=Forward  IdealPFdbkVariant=Disabled  SatFdbkVariant=Disabled  DerivativeFilterVariant=Disabled  NVariant=Disabled  NCopyVariant=Disabled_SignalSpec  FilterICVariant=Disabled  IntegratorICVariant=InternalICs  ExternalResetVariant=Disabled  TRSumVariant=Passthrough  SumFdbkVariant=Disabled  SumVariant=Passthrough_I  TsampFilterVariant=InternalTs  TsampNgainVariant=Passthrough  TsampIntegralVariant=Passthrough  ExternalSaturationOutDataTypeStr=Inherit: Same as second input
  Product2 : Product
  Sum1 : Sum  Inputs=|+-
  Sum2 : Sum  Inputs=|+-
  Sum5 : Sum  Inputs=|+-
  i* : Scope  NumInputPorts=2
  i*1 : Scope  NumInputPorts=2
  iq : Outport
  id : Outport  Port=2
  wires:
  P/1 -> Sum5/2
  Sum5/1 -> PID Controller4/1
  PID Controller4/1 -> Gain/1
  Sum1/1 -> PID Controller1/1
  Q_ref/1 -> Sum1/1
  Q/1 -> Sum1/2
  PID Controller1/1 -> Gain1/1
  Gain/1 -> iq/1, i*/1
  Gain1/1 -> id/1, i*/2
  V_DC/1 -> Sum2/2
  Constant/1 -> Sum2/1
  Sum2/1 -> PID Controller2/1
  PID Controller2/1 -> i*1/1, Product2/1
  Product2/1 -> Gain2/1
  Constant1/1 -> Product2/2
  P_ref/1 -> Sum5/1
  Gain2/1 -> i*1/2

== system MTDC_MODEL/GRID2+MMC2/Clarke Transformation  ==
  Constant : Constant  Value=0
  Constant1 : Constant  Value=1/2  SampleTime=0
  Constant2 : Constant  Value=1/2  SampleTime=0
  Constant3 : Constant  Value=1/2  SampleTime=0
  Constant4 : Constant  Value=2*pi/3  SampleTime=0
  Constant5 : Constant  SampleTime=0
  Constant6 : Constant  SampleTime=0
  Constant7 : Constant  SampleTime=0
  Gain7 : Gain  Gain=2/3
  Matrix Concatenate1 : Concatenate  NumInputs=3  Mode=Multidimensional array  ConcatenateDimension=2
  Matrix Concatenate2 : Concatenate  NumInputs=3  Mode=Multidimensional array  ConcatenateDimension=2
  Mux{1..6} (6 alike) : Mux  Inputs=3
  Sum1 : Sum  Inputs=|++
  Sum2 : Sum  Inputs=|+-
  Trigonometric Function : Trigonometry  Operator=cos
  Trigonometric Function1 : Trigonometry
  Trigonometric Function2 : Trigonometry  Operator=cos
  Trigonometric Function3 : Trigonometry
  Trigonometric Function4 : Trigonometry  Operator=cos
  Trigonometric Function5 : Trigonometry
  C : Outport  VectorParamsAs1DForOutWhenUnconnected=off
  "nC " : Outport  Port=2  VectorParamsAs1DForOutWhenUnconnected=off
  wires:
  Matrix Concatenate2/1 -> "nC "/1
  Gain7/1 -> C/1
  Constant/1 -> Trigonometric Function1/1, Trigonometric Function/1, Sum2/1, Sum1/1
  Mux6/1 -> Matrix Concatenate2/2
  Mux5/1 -> Matrix Concatenate2/1
  Matrix Concatenate1/1 -> Gain7/1
  Mux3/1 -> Matrix Concatenate1/3
  Mux1/1 -> Matrix Concatenate1/2
  Mux2/1 -> Matrix Concatenate1/1
  Trigonometric Function5/1 -> Mux3/2, Mux6/3
  Trigonometric Function4/1 -> Mux5/3, Mux3/1
  Trigonometric Function3/1 -> Mux1/2, Mux6/2
  Trigonometric Function2/1 -> Mux1/1, Mux5/2
  Trigonometric Function1/1 -> Mux6/1, Mux2/2
  Trigonometric Function/1 -> Mux5/1, Mux2/1
  Constant4/1 -> Sum1/2, Sum2/2
  Sum1/1 -> Trigonometric Function5/1, Trigonometric Function4/1
  Sum2/1 -> Trigonometric Function3/1, Trigonometric Function2/1
  Constant1/1 -> Mux2/3
  Constant2/1 -> Mux1/3
  Constant3/1 -> Mux3/3
  Constant5/1 -> Mux4/1
  Constant6/1 -> Mux4/2
  Constant7/1 -> Mux4/3
  Mux4/1 -> Matrix Concatenate2/3

== system MTDC_MODEL/GRID2+MMC2/Current loop1 ==
  note: Grid voltage qd frame
  Ref_iq : Inport
  Ref_id : Inport  Port=2
  iqd0 : Inport  Port=3
  vzqd0 : Inport  Port=4
  1SMC : Subsystem
  Constant2 : Constant  Value=2*pi*50  SampleTime=-1
  Constant3 : Constant  Value=0
  Current control d axis PI Controller : pid_lib/PID Controller  Controller=PI  Form=Parallel  TimeDomain=Continuous-time  UseExternalTs=off  SampleTime=1  IntegratorMethod=Forward Euler  FilterMethod=Forward Euler  ControllerParametersSource=internal  P=Kp_AC  I=Ki_AC  D=0  UseFilter=on  N=100  TunerSelectOption=Transfer Function Based (PID Tuner App)  InitialConditionSource=internal  InitialConditionForIntegrator=0  InitialConditionForFilter=0  DifferentiatorICPrevScaledInput=0  ExternalReset=none  TrackingMode=off  Kt=1  LimitOutput=off  SatLimitsSource=internal  UpperSaturationLimit=inf  LowerSaturationLimit=-inf  LinearizeAsGain=on  AntiWindupMode=none  Kb=1  POutMin=[]  POutMax=[]  IOutMin=[]  IOutMax=[]  DOutMin=[]  DOutMax=[]  NOutMin=[]  NOutMax=[]  SumOutMin=[]  SumOutMax=[]  SaturationOutMin=[]  SaturationOutMax=[]  PParamMin=[]  PParamMax=[]  IParamMin=[]  IParamMax=[]  DParamMin=[]  DParamMax=[]  NParamMin=[]  NParamMax=[]  KbParamMin=[]  KbParamMax=[]  KtParamMin=[]  KtParamMax=[]  KbOutMin=[]  KbOutMax=[]  KtOutMin=[]  KtOutMax=[]  IntegratorOutMin=[]  IntegratorOutMax=[]  FilterOutMin=[]  FilterOutMax=[]  SumI1OutMin=[]  SumI1OutMax=[]  SumI2OutMin=[]  SumI2OutMax=[]  SumI3OutMin=[]  SumI3OutMax=[]  SumI4OutMin=[]  SumI4OutMax=[]  SumDOutMin=[]  SumDOutMax=[]  DifferentiatorOutMin=[]  DifferentiatorOutMax=[]  FilterDiffOutCoefMin=[]  FilterDiffOutCoefMax=[]  ReciprocalOutMin=[]  ReciprocalOutMax=[]  SumDenOutMin=[]  SumDenOutMax=[]  SumNumOutMin=[]  SumNumOutMax=[]  DivideOutMin=[]  DivideOutMax=[]  UdiffTsProdOutMin=[]  UdiffTsProdOutMax=[]  NTsProdOutMin=[]  NTsProdOutMax=[]  UintegralTsProdOutMin=[]  UintegralTsProdOutMax=[]  UngainTsProdOutMin=[]  UngainTsProdOutMax=[]  IntegratorContinuousStateAttributes=''  IntegratorStateMustResolveToSignalObject=off  IntegratorRTWStateStorageClass=Auto  FilterContinuousStateAttributes=''  FilterStateMustResolveToSignalObject=off  FilterRTWStateStorageClass=Auto  ParallelPVariant=InternalParameters  IdealPVariant=Disabled  IVariant=InternalParameters  DVariant=Disabled  IntegratorVariant=Continuous  SatVariant=Disabled  AWVariant=Passthrough  PCopyVariant=Disabled  TRVariant=Disabled  FdbkBlocksVariant=Forward  IdealPFdbkVariant=Disabled  SatFdbkVariant=Disabled  DerivativeFilterVariant=Disabled  NVariant=Disabled  NCopyVariant=Disabled_SignalSpec  FilterICVariant=Disabled  IntegratorICVariant=InternalICs  ExternalResetVariant=Disabled  TRSumVariant=Passthrough  SumFdbkVariant=Disabled  SumVariant=Sum_PI  TsampFilterVariant=InternalTs  TsampNgainVariant=Passthrough  TsampIntegralVariant=Passthrough  ExternalSaturationOutDataTypeStr=Inherit: Same as second input
  Current control q axis PI Controller : pid_lib/PID Controller  Controller=PI  Form=Parallel  TimeDomain=Continuous-time  UseExternalTs=off  SampleTime=1  IntegratorMethod=Forward Euler  FilterMethod=Forward Euler  ControllerParametersSource=internal  P=Kp_AC  I=Ki_AC  D=0  UseFilter=on  N=100  TunerSelectOption=Transfer Function Based (PID Tuner App)  InitialConditionSource=internal  InitialConditionForIntegrator=0  InitialConditionForFilter=0  DifferentiatorICPrevScaledInput=0  ExternalReset=none  TrackingMode=off  Kt=1  LimitOutput=off  SatLimitsSource=internal  UpperSaturationLimit=inf  LowerSaturationLimit=-inf  LinearizeAsGain=on  AntiWindupMode=none  Kb=1  POutMin=[]  POutMax=[]  IOutMin=[]  IOutMax=[]  DOutMin=[]  DOutMax=[]  NOutMin=[]  NOutMax=[]  SumOutMin=[]  SumOutMax=[]  SaturationOutMin=[]  SaturationOutMax=[]  PParamMin=[]  PParamMax=[]  IParamMin=[]  IParamMax=[]  DParamMin=[]  DParamMax=[]  NParamMin=[]  NParamMax=[]  KbParamMin=[]  KbParamMax=[]  KtParamMin=[]  KtParamMax=[]  KbOutMin=[]  KbOutMax=[]  KtOutMin=[]  KtOutMax=[]  IntegratorOutMin=[]  IntegratorOutMax=[]  FilterOutMin=[]  FilterOutMax=[]  SumI1OutMin=[]  SumI1OutMax=[]  SumI2OutMin=[]  SumI2OutMax=[]  SumI3OutMin=[]  SumI3OutMax=[]  SumI4OutMin=[]  SumI4OutMax=[]  SumDOutMin=[]  SumDOutMax=[]  DifferentiatorOutMin=[]  DifferentiatorOutMax=[]  FilterDiffOutCoefMin=[]  FilterDiffOutCoefMax=[]  ReciprocalOutMin=[]  ReciprocalOutMax=[]  SumDenOutMin=[]  SumDenOutMax=[]  SumNumOutMin=[]  SumNumOutMax=[]  DivideOutMin=[]  DivideOutMax=[]  UdiffTsProdOutMin=[]  UdiffTsProdOutMax=[]  NTsProdOutMin=[]  NTsProdOutMax=[]  UintegralTsProdOutMin=[]  UintegralTsProdOutMax=[]  UngainTsProdOutMin=[]  UngainTsProdOutMax=[]  IntegratorContinuousStateAttributes=''  IntegratorStateMustResolveToSignalObject=off  IntegratorRTWStateStorageClass=Auto  FilterContinuousStateAttributes=''  FilterStateMustResolveToSignalObject=off  FilterRTWStateStorageClass=Auto  ParallelPVariant=InternalParameters  IdealPVariant=Disabled  IVariant=InternalParameters  DVariant=Disabled  IntegratorVariant=Continuous  SatVariant=Disabled  AWVariant=Passthrough  PCopyVariant=Disabled  TRVariant=Disabled  FdbkBlocksVariant=Forward  IdealPFdbkVariant=Disabled  SatFdbkVariant=Disabled  DerivativeFilterVariant=Disabled  NVariant=Disabled  NCopyVariant=Disabled_SignalSpec  FilterICVariant=Disabled  IntegratorICVariant=InternalICs  ExternalResetVariant=Disabled  TRSumVariant=Passthrough  SumFdbkVariant=Disabled  SumVariant=Sum_PI  TsampFilterVariant=InternalTs  TsampNgainVariant=Passthrough  TsampIntegralVariant=Passthrough  ExternalSaturationOutDataTypeStr=Inherit: Same as second input
  Demux1 : Demux  Outputs=2
  Demux2 : Demux  Outputs=2
  Divide : Product  Inputs=**
  Divide1 : Product  Inputs=**
  Gain1 : Gain  Gain=(Lg_1+La_1/2)
  Mux1 : Mux  Inputs=2
  Mux3 : Mux  Inputs=2
  Mux5 : Mux  Inputs=2
  PLCS : Subsystem
  SMC-Dynamic : Subsystem
  SMC1 : Subsystem
  ST-SMC : Subsystem
  Scope1 : Scope  NumInputPorts=2
  Scope2 : Scope
  Scope7 : Scope
  Sum3 : Sum  Inputs=-+|
  Sum4 : Sum  Inputs=|++
  Sum5 : Sum  Inputs=|+-
  Sum7 : Sum  Inputs=|+-
  Sum8 : Sum  Inputs=--|
  Twisting : Subsystem
  iqd0-iqd : Selector  InputPortWidth=3  IndexOptions=Index vector (dialog)  Indices=[1 2]  OutputSizes=1
  vzqd0-vzqd : Selector  InputPortWidth=3  IndexOptions=Index vector (dialog)  Indices=[1 2]  OutputSizes=1
  vlqd0 : Outport
  wires:
  Ref_iq/1 -> PLCS/2(Ref_iq), ST-SMC/2(Ref_iq), Twisting/2(Ref_iq), 1SMC/2(Ref_iq), SMC-Dynamic/2(Ref_iq), SMC1/3(Ref_iq), Sum5/1
  Ref_id/1 -> SMC1/2(Ref_id), PLCS/3(Ref_id), ST-SMC/3(Ref_id), Twisting/3(Ref_id), 1SMC/3(Ref_id), SMC-Dynamic/3(Ref_id), Sum3/2
  Current control q axis PI Controller/1 -> Sum8/1
  Mux3/1 -> Sum4/1
  vzqd0-vzqd/1 -> Demux1/1, Scope7/1, Sum4/2  "vzqd"
  Sum5/1 -> Current control q axis PI Controller/1
  Gain1/1 -> Divide1/1, Divide/2
  Constant2/1 -> Gain1/1
  Demux2/1 -> PLCS/1(iq), ST-SMC/1(iq), Twisting/1(iq), 1SMC/1(iq), SMC-Dynamic/1(iq), Divide1/2, Sum5/2
  Divide/1 -> Sum8/2
  vzqd0/1 -> vzqd0-vzqd/1  "vzqd0"
  Sum4/1 -> Mux5/1
  Sum3/1 -> Current control d axis PI Controller/1
  Divide1/1 -> Sum7/1
  Current control d axis PI Controller/1 -> Sum7/2
  Constant3/1 -> Mux5/2
  Demux2/2 -> Sum3/1, SMC1/1(id), Divide/1
  iqd0/1 -> iqd0-iqd/1
  iqd0-iqd/1 -> Demux2/1
  Sum8/1 -> Scope1/2
  SMC-Dynamic/2(Sq) -> [Sq]
  SMC1/2(Sd) -> [Sd]
  [Sq] -> Mux1/1
  [Sd] -> Mux1/2
  Mux1/1 -> Scope2/1
  Demux1/1 -> [vzq]
  [vzq] -> SMC-Dynamic/4(vzq)
  Mux5/1 -> vlqd0/1
  Sum7/1 -> Mux3/2
  1SMC/1(Out1) -> Scope1/1, Mux3/1

== system MTDC_MODEL/GRID2+MMC2/DC References ==
  Pt_DC : Inport
  Pab : Inport  Port=2
  Pac : Inport  Port=3
  Constant : Constant  Value=[1,1,1;1,-2,1;1,1,-2]
  Gain1 : Gain  Gain=1/(3*Vdc)
  Matrix Multiply2 : Product  Multiplication=Matrix(*)
  Mux10 : Mux  Inputs=3
  Sat3 : Subsystem
  isum_abc_ref_DC : Outport
  wires:
  Matrix Multiply2/1 -> Gain1/1
  Constant/1 -> Matrix Multiply2/1
  Mux10/1 -> Matrix Multiply2/2
  Gain1/1 -> Sat3/1(In1)  "isum_abc_ref_DC"
  Pt_DC/1 -> Mux10/1
  Pac/1 -> Mux10/3
  Pab/1 -> Mux10/2
  Sat3/1(Out1) -> isum_abc_ref_DC/1

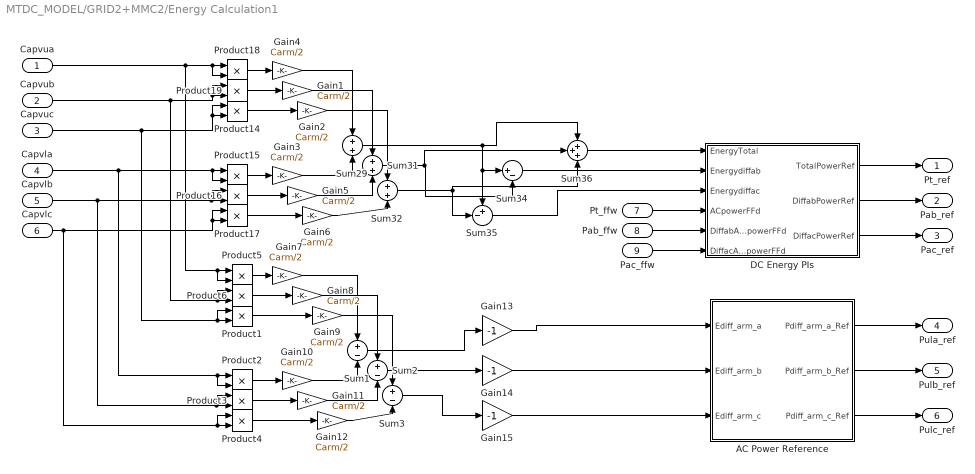
== system MTDC_MODEL/GRID2+MMC2/Energy Calculation1 ==
  Capvua : Inport
  Capvub : Inport  Port=2
  Capvuc : Inport  Port=3
  Capvla : Inport  Port=4
  Capvlb : Inport  Port=5
  Capvlc : Inport  Port=6
  Pt_ffw : Inport  Port=7
  Pab_ffw : Inport  Port=8
  Pac_ffw : Inport  Port=9
  AC Power Reference : Subsystem
  DC Energy PIs : Subsystem
  Gain{1..12} (12 alike) : Gain  Gain=Carm/2
  Gain13 : Gain  Gain=-1
  Gain14 : Gain  Gain=-1
  Gain15 : Gain  Gain=-1
  Product{1..6,14..19} (12 alike) : Product
  Sum1 : Sum  Inputs=+-
  Sum2 : Sum  Inputs=+-
  Sum29 : Sum
  Sum3 : Sum  Inputs=+-
  Sum31 : Sum
  Sum32 : Sum
  Sum34 : Sum  Inputs=|+-
  Sum35 : Sum  Inputs=+-|
  Sum36 : Sum  Inputs=+++
  Pt_ref : Outport
  Pab_ref : Outport  Port=2
  Pac_ref : Outport  Port=3
  Pula_ref : Outport  Port=4
  Pulb_ref : Outport  Port=5
  Pulc_ref : Outport  Port=6
  wires:
  Product6/1 -> Gain8/1
  Product4/1 -> Gain12/1
  Product2/1 -> Gain10/1
  Product1/1 -> Gain9/1
  Product3/1 -> Gain11/1
  Product5/1 -> Gain7/1
  Sum32/1 -> Sum36/3, Sum35/2
  Sum36/1 -> DC Energy PIs/1(EnergyTotal)
  Sum35/1 -> DC Energy PIs/3(Energydiffac)
  Sum34/1 -> DC Energy PIs/2(Energydiffab)
  Product19/1 -> Gain1/1
  Sum31/1 -> Sum36/2, Sum34/2
  Product17/1 -> Gain6/1
  Sum29/1 -> Sum35/1, Sum34/1, Sum36/1
  Product15/1 -> Gain3/1
  Product14/1 -> Gain2/1
  Product16/1 -> Gain5/1
  Product18/1 -> Gain4/1
  Capvlb/1 -> Product16/2, Product16/1, Product3/2, Product3/1
  Capvub/1 -> Product19/2, Product19/1, Product6/2, Product6/1
  Capvuc/1 -> Product14/2, Product14/1, Product1/2, Product1/1
  Capvua/1 -> Product18/1, Product18/2, Product5/1, Product5/2
  Capvla/1 -> Product15/1, Product15/2, Product2/1, Product2/2
  Capvlc/1 -> Product17/2, Product17/1, Product4/2, Product4/1
  Gain4/1 -> Sum29/1
  Gain1/1 -> Sum31/1
  Gain2/1 -> Sum32/1
  Gain9/1 -> Sum3/1
  Gain8/1 -> Sum2/1
  Gain7/1 -> Sum1/1
  Gain3/1 -> Sum29/2
  Gain5/1 -> Sum31/2
  Gain6/1 -> Sum32/2
  Gain10/1 -> Sum1/2
  Gain12/1 -> Sum3/2
  Gain11/1 -> Sum2/2
  Sum1/1 -> Gain13/1
  Sum2/1 -> Gain14/1
  Sum3/1 -> Gain15/1
  Pt_ffw/1 -> DC Energy PIs/4(ACpowerFFd)
  Pab_ffw/1 -> DC Energy PIs/5(DiffabABpowerFFd)
  Pac_ffw/1 -> DC Energy PIs/6(DiffacACpowerFFd)
  DC Energy PIs/1(TotalPowerRef) -> Pt_ref/1
  DC Energy PIs/3(DiffacPowerRef) -> Pac_ref/1
  DC Energy PIs/2(DiffabPowerRef) -> Pab_ref/1
  AC Power Reference/1(Pdiff_arm_a_Ref) -> Pula_ref/1
  AC Power Reference/2(Pdiff_arm_b_Ref) -> Pulb_ref/1
  AC Power Reference/3(Pdiff_arm_c_Ref) -> Pulc_ref/1
  Gain13/1 -> AC Power Reference/1(Ediff_arm_a)
  Gain15/1 -> AC Power Reference/3(Ediff_arm_c)
  Gain14/1 -> AC Power Reference/2(Ediff_arm_b)

== system MTDC_MODEL/GRID2+MMC2/Equivalent arm lower-a1 ==
  note: Power_la
  vla : Inport
  Controlled Current Source : spsControlledCurrentSourceLib/Controlled Current Source  Initialize=on  Source_Type=AC  Amplitude=0  Phase=0  Frequency=0  Measurements=None
  Controlled Voltage Source7 : spsControlledVoltageSourceLib/Controlled Voltage Source  Initialize=on  Source_Type=AC  Amplitude=Vdc/2  Phase=0  Frequency=0  Measurements=None
  Current Measurement4 : spsCurrentMeasurementLib/Current Measurement  PhasorSimulation=off  OutputType=Complex  PSBequivalent=0
  Divide1 : Product  Inputs=**
  Divide2 : Product  Inputs=*/
  Filtered Lower arm A instananeous power1 : Scope
  Gain : Gain  Gain=1e6
  Lower arm A instananeous power : Scope
  Series RLC Branch2 : spsSeriesRLCBranchLib/Series RLC Branch  LConnTagsString=__new0  RConnTagsString=__new0  BranchType=C  Resistance=Ra_1  Inductance=La_1  SetiL0=on  InitialCurrent=0  Capacitance=Cap/N  Setx0=on  InitialVoltage=640e3  Measurements=None
  Transfer Fcn : TransferFcn  Denominator=[1 1]
  Voltage Measurement : spsVoltageMeasurementLib/Voltage Measurement  PhasorSimulation=off  OutputType=Complex  PSBequivalent=0
  Conn1 : PMIOPort  Side=Right
  Conn2 : PMIOPort  Port=2  Side=Left
  v_sum_la : Outport
  wires:
  Gain/1 -> Filtered Lower arm A instananeous power1/1
  Transfer Fcn/1 -> Gain/1
  Current Measurement4/1 -> Divide1/2  "ila"
  Divide1/1 -> Divide2/1, Transfer Fcn/1, Lower arm A instananeous power/1
  Divide2/1 -> Controlled Current Source/1
  Voltage Measurement/1 -> Divide2/2, v_sum_la/1
  vla/1 -> Controlled Voltage Source7/1, Divide1/1  "vla"
  connections:
  Conn2/RConn1 -- Current Measurement4/RConn1
  Current Measurement4/LConn1 -- Controlled Voltage Source7/LConn1
  Voltage Measurement/LConn2 -- Series RLC Branch2/RConn1 -- Controlled Current Source/LConn1
  Controlled Current Source/RConn1 -- Series RLC Branch2/LConn1 -- Voltage Measurement/LConn1
  Controlled Voltage Source7/RConn1 -- Conn1/RConn1

== system MTDC_MODEL/GRID2+MMC2/Equivalent arm lower-a2 ==
  note: Power_lb
  vlb : Inport
  Controlled Current Source : spsControlledCurrentSourceLib/Controlled Current Source  Initialize=on  Source_Type=AC  Amplitude=0  Phase=0  Frequency=0  Measurements=None
  Controlled Voltage Source7 : spsControlledVoltageSourceLib/Controlled Voltage Source  Initialize=on  Source_Type=AC  Amplitude=Vdc/2  Phase=0  Frequency=0  Measurements=None
  Current Measurement4 : spsCurrentMeasurementLib/Current Measurement  PhasorSimulation=off  OutputType=Complex  PSBequivalent=0
  Divide1 : Product  Inputs=**
  Divide2 : Product  Inputs=*/
  Filtered Lower arm B instananeous power1 : Scope
  Gain : Gain  Gain=1e6
  Lower arm B instananeous power : Scope
  Series RLC Branch2 : spsSeriesRLCBranchLib/Series RLC Branch  LConnTagsString=__new0  RConnTagsString=__new0  BranchType=C  Resistance=Ra_1  Inductance=La_1  SetiL0=on  InitialCurrent=0  Capacitance=Cap/N  Setx0=on  InitialVoltage=640e3  Measurements=None
  Transfer Fcn : TransferFcn  Denominator=[1 1]
  Voltage Measurement : spsVoltageMeasurementLib/Voltage Measurement  PhasorSimulation=off  OutputType=Complex  PSBequivalent=0
  Conn1 : PMIOPort  Side=Right
  Conn2 : PMIOPort  Port=2  Side=Left
  v_sum_lb : Outport
  wires:
  vlb/1 -> Divide1/1, Controlled Voltage Source7/1  "vlb"
  Voltage Measurement/1 -> v_sum_lb/1, Divide2/2
  Divide2/1 -> Controlled Current Source/1
  Divide1/1 -> Lower arm B instananeous power/1, Transfer Fcn/1, Divide2/1
  Current Measurement4/1 -> Divide1/2  "ilb"
  Transfer Fcn/1 -> Gain/1
  Gain/1 -> Filtered Lower arm B instananeous power1/1
  connections:
  Controlled Voltage Source7/RConn1 -- Conn1/RConn1
  Voltage Measurement/LConn1 -- Series RLC Branch2/LConn1 -- Controlled Current Source/RConn1
  Controlled Current Source/LConn1 -- Series RLC Branch2/RConn1 -- Voltage Measurement/LConn2
  Current Measurement4/LConn1 -- Controlled Voltage Source7/LConn1
  Conn2/RConn1 -- Current Measurement4/RConn1
